simulink model "rangefinder_sim"  (R2024b)
settings: Solver=VariableStepAuto  StartTime=0.0  StopTime=30  RelTol=1e-3
undefined symbols (not defined in the file or in its folder): field_of_view, max_range, min_range, radiation_type, range
libraries: ros2lib x4
settings Model: Creator=DCHOME  LastModifiedBy=DCHOME

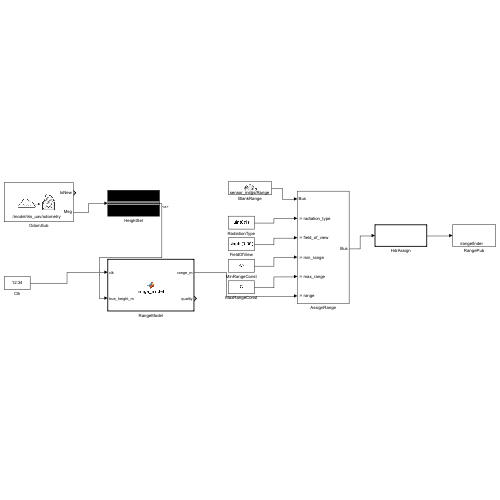
[thumbnail: Simulink's stored preview of the top-level diagram]
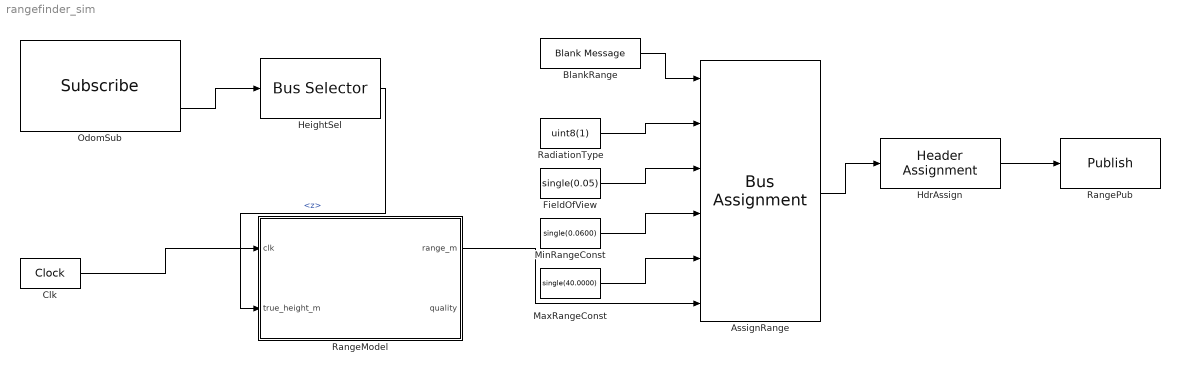
== system rangefinder_sim ==
  AssignRange : BusAssignment  AssignedSignals=radiation_type,field_of_view,min_range,max_range,range
  BlankRange : ros2lib/Blank Message  messageClass=Message  entityType=sensor_msgs/Range  messageType=sensor_msgs/Range  SampleTime=inf
  Clk : DigitalClock  SampleTime=0.1
  FieldOfView : Constant  Value=single(0.05)
  HdrAssign : ros2lib/Header Assignment  SetFrameID=on  FrameID=rangefinder  InsertTimeStamp=on  SetHeaderFieldName=Use the default header field name  HeaderFieldName=header
  HeightSel : BusSelector  OutputSignals=pose.pose.position.z
  MaxRangeConst : Constant  Value=single(40.0000)
  MinRangeConst : Constant  Value=single(0.0600)
  OdomSub : ros2lib/Subscribe  topicSource=Specify your own  topic=/model/iris_uav/odometry  messageType=nav_msgs/Odometry  sampleTime=0.1  QOSHistory=Keep last  QOSDepth=1  QOSReliability=Reliable  QOSDurability=Volatile  QOSDeadline=Inf  QOSLifespan=Inf  QOSLiveliness=Automatic  QOSLeaseDuration=Inf  QOSAvoidROSNamespaceConventions=off
  RadiationType : Constant  Value=uint8(1)
  RangeModel : MATLAB Function  TreatAsAtomicUnit=on
  RangePub : ros2lib/Publish  topicSource=Specify your own  topic=/rangefinder  messageType=sensor_msgs/Range  QOSHistory=Keep last  QOSDepth=1  QOSReliability=Reliable  QOSDurability=Volatile  QOSDeadline=Inf  QOSLifespan=Inf  QOSLiveliness=Automatic  QOSLeaseDuration=Inf  QOSAvoidROSNamespaceConventions=off
  wires:
  OdomSub/2 -> HeightSel/1
  Clk/1 -> RangeModel/1(clk)
  HeightSel/1 -> RangeModel/2(true_height_m)  "<z>"
  BlankRange/1 -> AssignRange/1
  RadiationType/1 -> AssignRange/2
  FieldOfView/1 -> AssignRange/3
  MinRangeConst/1 -> AssignRange/4
  MaxRangeConst/1 -> AssignRange/5
  RangeModel/1(range_m) -> AssignRange/6
  AssignRange/1 -> HdrAssign/1
  HdrAssign/1 -> RangePub/1

== matlab function rangefinder_sim/RangeModel ==
  data: clk input; range_m output; true_height_m input; quality output
function [range_m, quality] = range_model(clk, true_height_m)
    RANGE_MAX_M = 40.0000;
    RANGE_MIN_M = 0.0600;
    NOISE_STDDEV_FRAC = 0.0100;
    NOISE_STDDEV_BASE_M = 0.0200;
    DROPOUT_PROB = 0.1500;
    true_height_m = max(true_height_m, 0);
    noise_sigma = NOISE_STDDEV_BASE_M + NOISE_STDDEV_FRAC * true_height_m;
    noisy = true_height_m + noise_sigma * randn();
    if rand() < DROPOUT_PROB || true_height_m > RANGE_MAX_M || true_height_m < RANGE_MIN_M
        % Dropout / out-of-range: sensor reports max range with zero quality,
        % matching how real rangefinders signal 'no valid return'.
        range_m = single(RANGE_MAX_M);
        quality = uint8(0);
    else
        range_m = single(min(max(noisy, RANGE_MIN_M), RANGE_MAX_M));
        quality = uint8(200 + round(randn() * 20));
    end
end
